simulink model "CurveHighVel"  (R2024b)
settings: Solver=VariableStepAuto  StartTime=0.0  StopTime=Ts  RelTol=1e-3
PreLoadFcn:
  | setUpCurveHighVel
model workspace (MAT data in the model file):
  firstWarning = 0
  originalScenarioChecksum = 'F73A6DA3C723D3CA73A6F931B7A52A9C'
values from neighbouring files (symbols this model uses):
  K = lqr(A,B,Q,R)    [LQR_Coeff_High_Vel.m]
  m = 2000    [LQR_Coeff_High_Vel.m]
  psi_o = 0    [setUpCurveHighVel.m]
  s = size(xRef)    [setUpCurveHighVel.m]
  vel = lookUpt(2:30,2:20)    [setUpCurveHighVel.m]
  X_o = refPose(1,1)    [setUpCurveHighVel.m]
  xlt = lookUpt(2:30,1)    [setUpCurveHighVel.m]
  xRef = refPose(:,1)    [setUpCurveHighVel.m]
  Y_o = -refPose(1,2)    [setUpCurveHighVel.m]
  ylt = lookUpt(1,2:20)    [setUpCurveHighVel.m]
  yRef = -refPose(:,2)    [setUpCurveHighVel.m]
libraries: simulink x5, autolibutils x4, autolibshared x3, slpidlib x2, vehdynlibviscommon x1
(part 3 of 3)

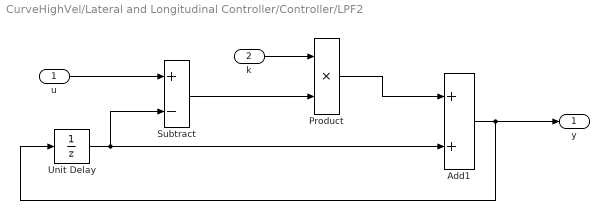
== system CurveHighVel/Lateral and Longitudinal Controller/Controller/LPF2 ==
  u : Inport
  k : Inport  Port=2
  Add1 : Sum
  Product : Product
  Subtract : Sum  Inputs=+-
  Unit Delay : UnitDelay  SampleTime=-1  HasFrameUpgradeWarning=on
  y : Outport
  wires:
  k/1 -> Product/1
  Product/1 -> Add1/1
  Add1/1 -> y/1, Unit Delay/1
  Unit Delay/1 -> Subtract/2, Add1/2
  u/1 -> Subtract/1
  Subtract/1 -> Product/2

== system CurveHighVel/Lateral and Longitudinal Controller/Controller/LPF3 ==
  u : Inport
  k : Inport  Port=2
  Add1 : Sum
  Product : Product
  Subtract : Sum  Inputs=+-
  Unit Delay : UnitDelay  SampleTime=-1  HasFrameUpgradeWarning=on
  y : Outport
  wires:
  k/1 -> Product/1
  Product/1 -> Add1/1
  Add1/1 -> y/1, Unit Delay/1
  Unit Delay/1 -> Subtract/2, Add1/2
  u/1 -> Subtract/1
  Subtract/1 -> Product/2

== system CurveHighVel/Powertrain & Driveline/Driveline/AWD ==
  TPowertrain : Inport
  AWD : Gain  Gain=[1;1;1;1]./2
  TAxles : Outport  VectorParamsAs1DForOutWhenUnconnected=off
  wires:
  TPowertrain/1 -> AWD/1
  AWD/1 -> TAxles/1

== system CurveHighVel/Powertrain & Driveline/Driveline/FWD ==
  TPowertrain : Inport
  FWD : Gain  Gain=[1;1;0;0]
  TAxles : Outport  VectorParamsAs1DForOutWhenUnconnected=off
  wires:
  FWD/1 -> TAxles/1
  TPowertrain/1 -> FWD/1

== system CurveHighVel/Powertrain & Driveline/Driveline/RWD ==
  TPowertrain : Inport
  RWD : Gain  Gain=[0;0;1;1]
  TAxles : Outport  VectorParamsAs1DForOutWhenUnconnected=off
  wires:
  TPowertrain/1 -> RWD/1
  RWD/1 -> TAxles/1

== matlab function CurveHighVel/Lateral and Longitudinal Controller/Controller/MATLAB Function ==
  data: pose input; e output; way_point input; v input; cte output; yaw_ref output
function [e,cte,yaw_ref]= error(pose,way_point,v)

    x = pose(1);
    y = pose(2);
    yaw = pose(3);

    nearest_idx = find_nearest_waypoint(x,y,way_point);
    [cte,heading_error,yaw_ref]= compute_cte(x,y,yaw,way_point,nearest_idx,v);    



e = heading_error;
end


function idx = find_nearest_waypoint(x, y, waypoints)
    dists = vecnorm((waypoints - [x, y]).');
    [~, idx] = min(dists);
end
 
function [cte,heading_error,yaw_ref] = compute_cte(x,y,yaw,way_point,idx,v)
    wp1 = way_point(idx,:);
    wp1 = wp1';

    if idx < size(way_point,1)
        wp2 = way_point(idx+1,:);
    else
        wp2 = wp1;
    end
    wp2 = wp2';


    dx = wp2(1) - wp1(1);
    dy = wp2(2) - wp1(2);

    target_angle = atan2(dy, dx);
    heading_error = target_angle - yaw;
    % if heading_error > pi
    %     heading_error = heading_error - 2 * pi;
    % elseif heading_error < -pi
    %     heading_error = heading_error + 2 * pi;
    % end
     

    cte = -sin(yaw) * dx + cos(yaw) * dy;
    cte = v*sin(yaw + heading_error);

    

    seg_vec = [dx,dy];
    pos_vec = [x-wp1(1),y-wp1(2)];
    cross_val = dx * pos_vec(2) - dy * pos_vec(1);
    seg_len = norm(seg_vec) + 1e-6;
    cte = (cross_val / seg_len);
    heading_error = rem(heading_error+pi,2*pi) - pi;
    yaw_ref = target_angle;


    
end

== matlab function CurveHighVel/Lateral and Longitudinal Controller/Controller/MATLAB Function1 ==
  data: cte input; heading_error input; v input; pose input; u output; heading_error_rate input; yawrate_ref input; cte_dot input; K input
function u = lqr(cte,heading_error,v,pose,heading_error_rate,yawrate_ref,cte_dot,K)

    x = pose(1);
    y = pose(2);
    yaw = pose(3);
    Iz = 4000; %kg*m^2
    la = 1.4; %m
    lb = 1.6; %4
    h = 0.35; %m
    m = 2000; %m
    tw = 1.4; %m
    Cf = 2*12000; % N/rad
    Cr = 2*11000; %N/rad
    v = 10;

    
    % cte_dot = v*cos(yaw)*heading_error + v*sin(yaw);
    e_vec = [cte,cte_dot,heading_error,heading_error_rate]';
    
    u = (K(1)*e_vec(1)+K(2)*e_vec(2)+K(3)*e_vec(3)+K(4)*e_vec(4))+heading_error+0.001*yawrate_ref*(la+lb)/10;

 


    

end

== matlab function CurveHighVel/Lateral and Longitudinal Controller/Controller/MATLAB Function2 ==
  data: cte input; heading_error input; v input; pose input; u output; heading_error_rate input; yawrate_ref input; cte_dot input; K1 input; K2 input
function u = smc(cte,heading_error,v,pose,heading_error_rate,yawrate_ref,cte_dot,K1,K2)

    x = pose(1);
    y = pose(2);
    yaw = pose(3);
    Iz = 4000; %kg*m^2
    la = 1.4; %m
    lb = 1.6; %4
    h = 0.35; %m
    m = 2000; %m
    tw = 1.4; %m
    Cf = 2*12000; % N/rad
    Cr = 2*11000; %N/rad
    v = 10;
    temp2 = -(Cf + Cr)/m;
    temp1 = -(Cf*la - Cr*lb);
    temp3 = -(Cf*la^2 + Cr*lb^2)/v/Iz;



    
    % cte_dot = v*cos(yaw)*heading_error + v*sin(yaw);
    e_vec = [cte,cte_dot,heading_error,heading_error_rate]';

    c1 = 0.07;
    c2 = 0.0005;

    s = c1*cte_dot + c2*heading_error;
    
    u = -m*(-(temp1/m/v - v)*yawrate_ref - temp2*cte_dot/v + temp2*heading_error - temp2*(heading_error_rate)/m/v - K1 *tanh(s) - c2*heading_error_rate/c1 - K2*s )/Cf;

    

end

== matlab function CurveHighVel/Lateral and Longitudinal Controller/Controller/MATLAB Function3 ==
  data: cte input; heading_error input; v input; pose input; u output; heading_error_rate input; yawrate_ref input; cte_dot input; k input
function u  = mrac(cte,heading_error,v,pose,heading_error_rate,yawrate_ref,cte_dot,k)


    x = pose(1);
    y = pose(2);
    yaw = pose(3);
    
    Iz = 4000; %kg*m^2
    la = 1.4; %m
    lb = 1.6; %4
    h = 0.35; %m
    m = 2000; %m
    tw = 1.4; %m
    Cf = 2*12000; % N/rad
    Cr = 2*11000; %N/rad

    % 


    % cte_dot = v*cos(yaw)*heading_error + v*sin(yaw);
        c2 = (Cf*la - Cr*lb)/Iz;
        c1 = -c2/v;
        c3 = -(Cf*la^2 + Cr*lb^2)/Iz/v;
    
        u = -m*(k*heading_error_rate + c1*cte_dot + c2*heading_error + c3*heading_error_rate + c3*yawrate_ref)/Cf;








end
